simulink model "Tunnel_heist"  (R2020a)
settings: Solver=FixedStepDiscrete  StartTime=0.0  StopTime=15  FixedStep=1  RelTol=1e-3
values from neighbouring files (symbols this model uses):
  Ignition : value not decoded    [ALS_Project_dd.sldd]
  Tunnel_detected : value not decoded    [ALS_Project_dd.sldd]
undefined symbols (not defined in the file or in its folder): AlsMode, Headlights, sigbuilder_block, Visuallights
libraries: simulink x8
settings Model: DataDictionary=data_tunnel.sldd  Creator=Amol Madhukar Patil  LastModifiedBy=hp
settings OptimizationCC: DefaultParameterBehavior=Inlined  EnhancedBackFolding=on  PassReuseOutputArgsAs=Individual arguments  OptimizeBlockOrder=speed  DifferentSizesBufferReuse=on  OptimizationCustomize=off  EfficientTunableParamExpr=on
settings DebuggingCC: SignalInfNanChecking=error  ParameterTunabilityLossMsg=error  UniqueDataStoreMsg=warning  StrictBusMsg=ErrorOnBusTreatedAsVector
settings SFSimCC: MATLABDynamicMemAlloc=off  CustomCodeUndefinedFunction=UseInterfaceOnly
settings RTWCC: SystemTargetFile=ert.tlc  GenCodeOnly=on  TemplateMakefile=ert_default_tmf  GenerateReport=on  IncludeHyperlinkInReport=on  LaunchReport=on  GenerateTraceInfo=on  GenerateTraceReport=on  GenerateTraceReportSl=on  GenerateTraceReportSf=on  GenerateTraceReportEml=on
settings CodeAppCC: ForceParamTrailComments=on  IgnoreCustomStorageClasses=off  OperatorAnnotations=on  SimulinkDataObjDesc=on  SFDataObjDesc=on  InsertBlockDesc=on
settings ERTTargetCC: TargetLangStandard=C99 (ISO)  GenerateSampleERTMain=on  InlinedParameterPlacement=NonHierarchical  ERTCustomFileTemplate=example_file_process.tlc
settings ConfigComp: CovMetricSettings=dcmswe

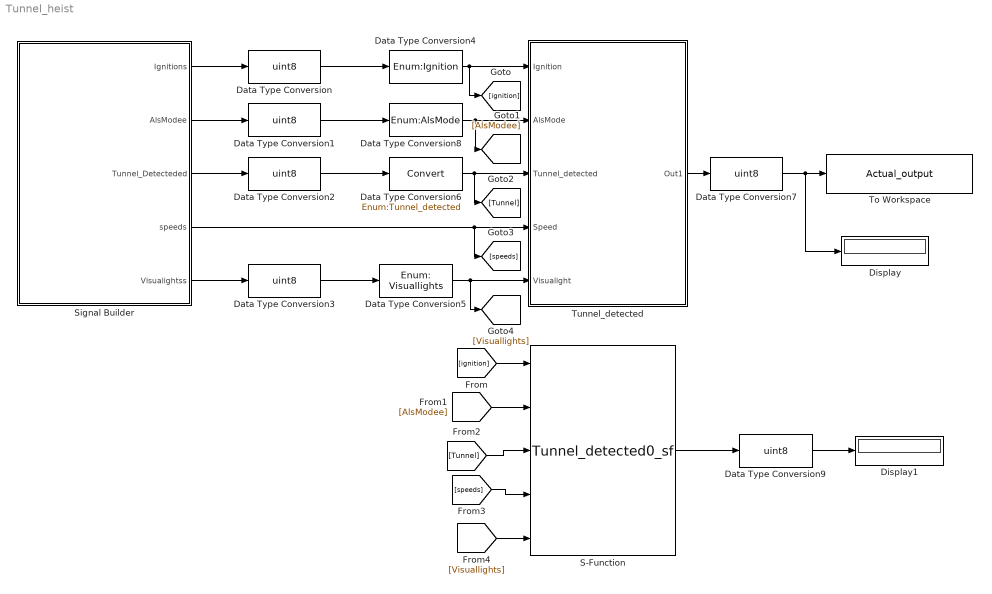
== system Tunnel_heist ==
  Data Type Conversion{,1..2,7,9} (5 alike) : DataTypeConversion  OutDataTypeStr=uint8  SaturateOnIntegerOverflow=on  LockScale=on
  Data Type Conversion3 : DataTypeConversion  OutDataTypeStr=uint8  LockScale=on
  Data Type Conversion4 : DataTypeConversion  OutDataTypeStr=Enum:Ignition  SaturateOnIntegerOverflow=on  LockScale=on
  Data Type Conversion5 : DataTypeConversion  OutDataTypeStr=Enum: Visuallights  SaturateOnIntegerOverflow=on  LockScale=on
  Data Type Conversion6 : DataTypeConversion  OutDataTypeStr=Enum:Tunnel_detected  SaturateOnIntegerOverflow=on  LockScale=on
  Data Type Conversion8 : DataTypeConversion  OutDataTypeStr=Enum:AlsMode  SaturateOnIntegerOverflow=on  LockScale=on
  Display : Display
  Display1 : Display
  S-Function : S-Function  FunctionName=Tunnel_detected0_sf  SFunctionDeploymentMode=off  EnableBusSupport=off
  Signal Builder : Subsystem  Tag=STV Subsys  LoadFcn=sigbuilder_block('load');  StartFcn=sigbuilder_block('start');  StopFcn=sigbuilder_block('stop');  ClipboardFcn=sigbuilder_block('clipboard');  mask(Sigbuilder block){tuvar=[0:10]}
      mask help: Simulink:masks:SigbuilderBlock_MD
      mask init:
      | if ~strcmp(get_param(bdroot(gcbh),'SimulationStatus'),'stopped') tuvar = sigbuilder_block('maskInit'); end
      settings: CopyFcn=sigbuilder_block('copy');  DeleteFcn=sigbuilder_block('delete');  ModelCloseFcn=sigbuilder_block('modelClose');  PreSaveFcn=sigbuilder_block('preSave');  PauseFcn=sigbuilder_block('pause');  ContinueFcn=sigbuilder_block('continue');  NameChangeFcn=sigbuilder_block('namechange');  OpenFcn=sigbuilder_block('open',[440.25 156.75 544.5 355.5 ]);  CloseFcn=sigbuilder_block('close');
      mask Display: plot(0, 0, 100, 100,[2, 2, 32, 32, 2], [68, 8, 8, 68, 68],[32, 2], [38, 38], [32, 19, 2],[53, 60, 44], [32, 17, 17, 2],[16, 16, 31, 31]);txt = getActiveGroup(gcbh);text(2, 100, txt,'verticalAlignment', 'top');
  To Workspace : ToWorkspace  VariableName=Actual_output  SaveFormat=Timeseries  SampleTime=-1
  "Tunnel_detected " : Subsystem  TreatAsAtomicUnit=on
  wires:
  "Tunnel_detected "/1(Out1) -> Data Type Conversion7/1
  Data Type Conversion/1 -> Data Type Conversion4/1
  Data Type Conversion1/1 -> Data Type Conversion8/1
  Data Type Conversion2/1 -> Data Type Conversion6/1
  Data Type Conversion4/1 -> [ignition], "Tunnel_detected "/1(Ignition)
  Data Type Conversion8/1 -> [AlsModee], "Tunnel_detected "/2(AlsMode)
  Data Type Conversion6/1 -> [Tunnel], "Tunnel_detected "/3(Tunnel_detected)
  Data Type Conversion3/1 -> Data Type Conversion5/1
  Signal Builder/1(Ignitions) -> Data Type Conversion/1
  Signal Builder/2(AlsModee) -> Data Type Conversion1/1
  Signal Builder/3(Tunnel_Detecteded) -> Data Type Conversion2/1
  Signal Builder/5(Visualightss) -> Data Type Conversion3/1
  Signal Builder/4(speeds) -> [speeds], "Tunnel_detected "/4(Speed)
  Data Type Conversion5/1 -> [Visuallights], "Tunnel_detected "/5(Visualight)
  Data Type Conversion7/1 -> Display/1, To Workspace/1
  [ignition] -> S-Function/1
  [AlsModee] -> S-Function/2
  [Tunnel] -> S-Function/3
  [speeds] -> S-Function/4
  [Visuallights] -> S-Function/5
  S-Function/1 -> Data Type Conversion9/1
  Data Type Conversion9/1 -> Display1/1

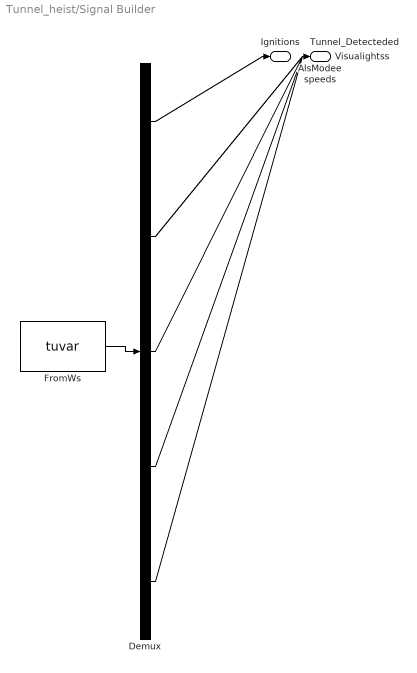
== system Tunnel_heist/Signal Builder ==
  Demux : Demux  Tag=STV Demux  Outputs=5
      settings: DisplayOption=none
  FromWs : FromWorkspace  Tag=STV FromWs  VariableName=tuvar
      SigBuilderData=|
      | common.afterFinalStr = 'Extrapolate'
      | common.sampleTime = 0
      | dataSet.timeRange = [0 10]
      | dataSet.name = 'Sheet1'
      | sbobj.Groups.Name = 'Sheet1'
      | sbobj.Groups.Signals(1).Name = 'Ignitions'
      | sbobj.Groups.Signals(1).XData = [0 1 2 3 4 5 6 7 8 9 10]
      | sbobj.Groups.Signals(1).YData = [1 0 1 1 1 1 1 1 0 1 1]
      | sbobj.Groups.Signals(2).Name = 'AlsModee'
      | sbobj.Groups.Signals(2).XData = [0 1 2 3 4 5 6 7 8 9 10]
      | sbobj.Groups.Signals(2).YData = [0 1 0 0 0 0 0 0 0 0 1]
      | sbobj.Groups.Signals(3).Name = 'Tunnel_Detecteded'
      | sbobj.Groups.Signals(3).XData = [0 1 2 3 4 5 6 7 8 9 10]
      | sbobj.Groups.Signals(3).YData = [0 0 1 0 0 0 0 0 0 1 0]
      | sbobj.Groups.Signals(4).Name = 'speeds'
      | sbobj.Groups.Signals(4).XData = [0 1 2 3 4 5 6 7 8 9 10]
      | sbobj.Groups.Signals(4).YData = [30 23 17 26 43 34 39 78 28 54 65]
      | sbobj.Groups.Signals(5).Name = 'Visualightss'
      | sbobj.Groups.Signals(5).XData = [0 1 2 3 4 5 6 7 8 9 10]
      | sbobj.Groups.Signals(5).YData = [0 0 0 0 0 0 0 0 0 0 0]
  Ignitions : Outport  Tag=STV Outport  VectorParamsAs1DForOutWhenUnconnected=off
  AlsModee : Outport  Tag=STV Outport  Port=2  VectorParamsAs1DForOutWhenUnconnected=off
  Tunnel_Detecteded : Outport  Tag=STV Outport  Port=3  VectorParamsAs1DForOutWhenUnconnected=off
  speeds : Outport  Tag=STV Outport  Port=4  VectorParamsAs1DForOutWhenUnconnected=off
  Visualightss : Outport  Tag=STV Outport  Port=5  VectorParamsAs1DForOutWhenUnconnected=off
  wires:
  FromWs/1 -> Demux/1
  Demux/1 -> Ignitions/1
  Demux/2 -> AlsModee/1
  Demux/3 -> Tunnel_Detecteded/1
  Demux/4 -> speeds/1
  Demux/5 -> Visualightss/1

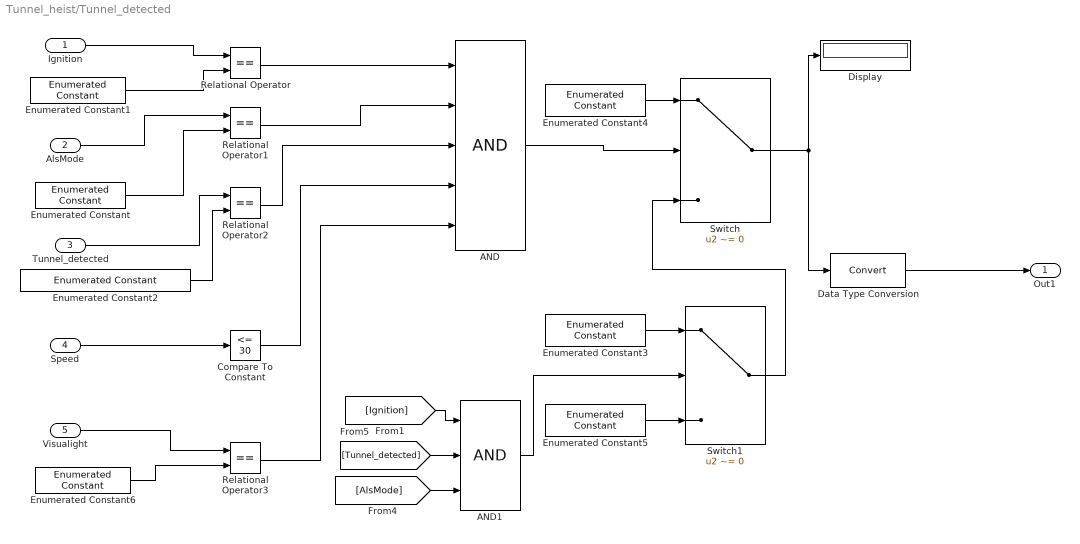
== system Tunnel_heist/Tunnel_detected  ==
  Ignition : Inport
  AlsMode : Inport  Port=2
  Tunnel_detected : Inport  Port=3
  Speed : Inport  Port=4
  Visualight : Inport  Port=5
  AND : Logic  Inputs=5  AllPortsSameDT=off  OutDataTypeStr=boolean
  AND1 : Logic  Inputs=3  AllPortsSameDT=off  OutDataTypeStr=boolean
  Compare To Constant : simulink/Logic and Bit Operations/Compare To Constant  relop=<=  const=30  OutDataTypeStr=uint8
  Data Type Conversion : DataTypeConversion
  Display : Display
  Enumerated Constant : simulink/Sources/Enumerated Constant  OutDataTypeStr=Enum: AlsMode  Value=AlsMode.On  SampleTime=inf
  Enumerated Constant1 : simulink/Sources/Enumerated Constant  OutDataTypeStr=Enum: Ignition  Value=Ignition.Ignition_On  SampleTime=inf
  Enumerated Constant2 : simulink/Sources/Enumerated Constant  OutDataTypeStr=Enum: Tunnel_detected  Value=Tunnel_detected.tunnel_detected_On  SampleTime=inf
  Enumerated Constant3 : simulink/Sources/Enumerated Constant  OutDataTypeStr=Enum: Headlights  Value=Headlights.Highbeam  SampleTime=inf
  Enumerated Constant4 : simulink/Sources/Enumerated Constant  OutDataTypeStr=Enum: Headlights  Value=Headlights.Lowbeam  SampleTime=inf
  Enumerated Constant5 : simulink/Sources/Enumerated Constant  OutDataTypeStr=Enum: Headlights  Value=Headlights.Headlight_Off  SampleTime=inf
  Enumerated Constant6 : simulink/Sources/Enumerated Constant  OutDataTypeStr=Enum: Visuallights  Value=Visuallights.nighttime  SampleTime=inf
  Relational Operator{,1..3} (4 alike) : RelationalOperator  Operator===  OutDataTypeStr=boolean  RndMeth=Simplest
  Switch : Switch  Criteria=u2 ~= 0
  Switch1 : Switch  Criteria=u2 ~= 0
  Out1 : Outport  VectorParamsAs1DForOutWhenUnconnected=off
  wires:
  [AlsMode] -> AND1/3
  [Tunnel_detected] -> AND1/2
  [Ignition] -> AND1/1
  Ignition/1 -> Relational Operator/1
  Switch1/1 -> Switch/3
  Enumerated Constant3/1 -> Switch1/1
  Enumerated Constant5/1 -> Switch1/3
  Enumerated Constant1/1 -> Relational Operator/2
  Enumerated Constant6/1 -> Relational Operator3/2
  Enumerated Constant/1 -> Relational Operator1/2
  Enumerated Constant2/1 -> Relational Operator2/2
  Enumerated Constant4/1 -> Switch/1
  AND1/1 -> Switch1/2
  AlsMode/1 -> Relational Operator1/1
  AND/1 -> Switch/2
  Tunnel_detected/1 -> Relational Operator2/1
  Switch/1 -> Display/1, Data Type Conversion/1
  Speed/1 -> Compare To Constant/1
  Visualight/1 -> Relational Operator3/1
  Data Type Conversion/1 -> Out1/1
  Relational Operator/1 -> AND/1
  Relational Operator1/1 -> AND/2
  Relational Operator2/1 -> AND/3
  Compare To Constant/1 -> AND/4
  Relational Operator3/1 -> AND/5
